simulink model "zadanie3"  (R2023b)
settings: Solver=FixedStepAuto  StartTime=0.0  StopTime=200  FixedStep=0.0001  RelTol=1e-3
values from neighbouring files (symbols this model uses):
  c_denom = [ 1, 3, 3, 1]    [Copy_of_zadanie2.m]    (also in laboratorium5.m = [ 1, 3, 2]; zadanie2.m)
  c_nom = [ 0, 0, 0, 1 ]    [Copy_of_zadanie2.m]    (also in laboratorium5.m = [ 0, 0, 1 ]; zadanie2.m)
  final_value = 1    [Copy_of_zadanie2.m]    (also in laboratorium5.m; zadanie2.m)
  init_value = 0    [Copy_of_zadanie2.m]    (also in laboratorium5.m; zadanie2.m)
  pi_cont_denom = [ 1, 0]    [Copy_of_zadanie2.m]    (also in zadanie2.m)
  pi_cont_nom = [ kp, ki ]    [Copy_of_zadanie2.m]    (also in zadanie2.m)
  time_step = 0    [Copy_of_zadanie2.m]    (also in laboratorium5.m; zadanie2.m)
settings Model: Creator=student  LastModifiedBy=tomasz
settings SolverCC: AlgebraicLoopSolver=TrustRegion
settings DebuggingCC: UnconnectedInputMsg=warning  UnconnectedOutputMsg=warning  UnconnectedLineMsg=warning
settings ModelReferenceCC: EnableRefExpFcnMdlSchedulingChecks=on
settings RTWCC: DLArmComputeVersion=19.05

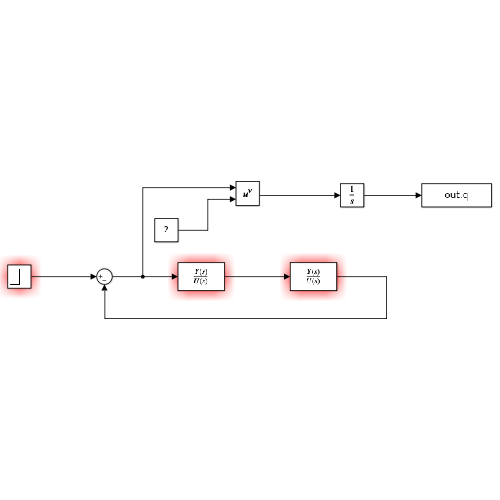
[thumbnail: Simulink's stored preview of the top-level diagram]
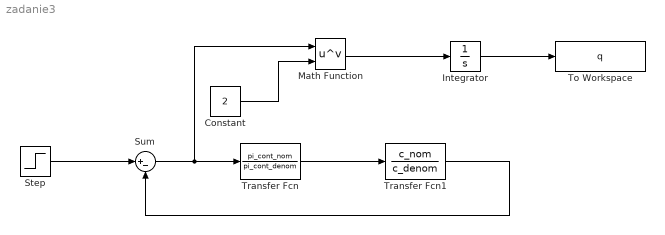
== system zadanie3 ==
  Constant : Constant  Value=2
  Integrator : Integrator
  Math Function : Math  Operator=pow
  Step : Step  Time=time_step  Before=init_value  After=final_value  SampleTime=0
  Sum : Sum  Inputs=|+-
  To Workspace : ToWorkspace  VariableName=q  SaveFormat=Timeseries  SampleTime=-1
  Transfer Fcn : TransferFcn  Numerator=pi_cont_nom  Denominator=pi_cont_denom
  Transfer Fcn1 : TransferFcn  Numerator=c_nom  Denominator=c_denom
  wires:
  Step/1 -> Sum/1
  Sum/1 -> Transfer Fcn/1, Math Function/1
  Transfer Fcn1/1 -> Sum/2
  Math Function/1 -> Integrator/1
  Constant/1 -> Math Function/2
  Integrator/1 -> To Workspace/1
  Transfer Fcn/1 -> Transfer Fcn1/1
